simulink model "verify_Wall_in_mdl"  (R2016b)
settings: Solver=ode45  StartTime=0  StopTime=24*3600  MaxStep=100  RelTol=1e-3  EnableMultiTasking=on
libraries: carnot x5
settings Model: Creator=drhf  LastModifiedBy=User
settings DataIOCC: SaveFormat=Array  SignalLoggingSaveFormat=ModelDataLogs
settings OptimizationCC: ExpressionDepthLimit=2147483647  LifeSpan=inf
settings DebuggingCC: UnderspecifiedInitializationDetection=Classic  MergeDetectMultiDrivingBlocksExec=none  SolverPrmCheckMsg=warning  FcnCallInpInsideContextMsg=warning  StateNameClashWarn=warning  SFUnexpectedBacktrackingDiag=warning  SFNoUnconditionalDefaultTransitionDiag=warning  SFExecutionAtInitializationDiag=none
settings HardwareCC: ProdBitPerPointer=32  ProdBitPerSizeT=32  ProdBitPerPtrDiffT=32  ProdLargestAtomicFloat=None  ProdIntDivRoundTo=Undefined  ProdEndianess=Unspecified  ProdWordSize=32  ProdHWDeviceType=32-bit Generic
settings ModelReferenceCC: PropagateSignalLabelsOutOfModel=off
settings GRTTargetCC: TargetLangStandard=C89/C90 (ANSI)  GeneratePreprocessorConditionals=Disable all  CombineOutputUpdateFcns=off  GRTInterface=on
settings ConfigComp: CovMetricSettings=dw  CovHtmlReporting=on  CovSaveCumulativeToWorkspaceVar=on  CovSaveSingleToWorkspaceVar=on  CovExternalEMLEnable=off

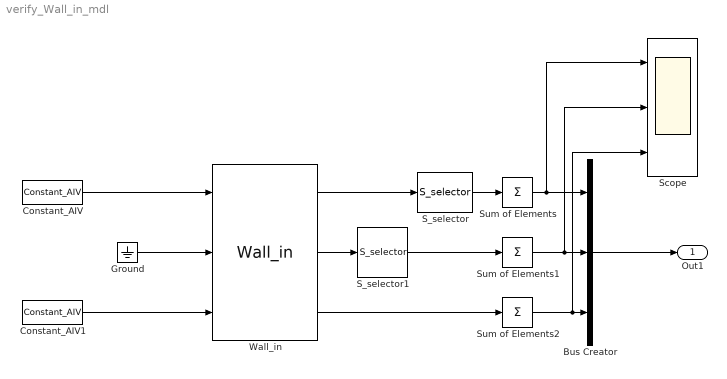
== system verify_Wall_in_mdl ==
  Bus Creator : BusCreator  Inputs=3
  Constant_AIV : carnot/Source/Ventilation/Constant_AIV  Tsens=20  Tcon=20  Trad=20  mw=0.012  mco=0.01  rhoair=1.2  cpair=1004  pair=100000  nair=0.5
  Constant_AIV1 : carnot/Source/Ventilation/Constant_AIV  Tsens=10  Tcon=10  Trad=10  mw=0.012  mco=0.01  rhoair=1.2  cpair=1004  pair=100000  nair=0.5
  Ground : Ground
  S_selector : carnot/Outputs/S_selector  e1=off  e2=off  e3=off  e4=off  e5=off  e6=off  e7=on  e8=on  e9=off  e10=off  e11=off  e12=off  e13=off
  S_selector1 : carnot/Outputs/S_selector  e1=off  e2=off  e3=off  e4=off  e5=off  e6=off  e7=on  e8=on  e9=off  e10=off  e11=off  e12=off  e13=off
  Scope : Scope  NumInputPorts=3
  Sum of Elements : Sum  Inputs=+
  Sum of Elements1 : Sum  Inputs=+
  Sum of Elements2 : Sum  Inputs=+
  Wall_in : carnot/Load/Houses/wall_floor/Wall_in  wallsize=[10 10]  d=[0.1 0.1 0.1]  cond=[1 1 1]  cwall=[0.28 0.28 0.28]*3600  rho=[2000 200 2000]  emission_in=.96  dactive=[0.075 0.15 0.225]  t0=10  tau=10*3600
  Out1 : Outport
  wires:
  Bus Creator/1 -> Out1/1
  Wall_in/1 -> S_selector/1
  Constant_AIV/1 -> Wall_in/1
  Constant_AIV1/1 -> Wall_in/3
  Ground/1 -> Wall_in/2
  S_selector/1 -> Sum of Elements/1
  Wall_in/2 -> S_selector1/1
  Sum of Elements/1 -> Scope/1, Bus Creator/1
  Wall_in/3 -> Sum of Elements2/1
  Sum of Elements1/1 -> Scope/2, Bus Creator/2
  S_selector1/1 -> Sum of Elements1/1
  Sum of Elements2/1 -> Scope/3, Bus Creator/3
